simulink subsystem "rss_StrtUpElecAgCalcNeed"  (R2023a)
settings: Solver=VariableStepAuto  StartTime=0.0  StopTime=10.0  RelTol=1e-3
undefined symbols (not defined in the file): Cdbl_nElecAgSpdMaxVal, Cdbl_nElecAgSpdPeakVal, Cdbl_tiMedTaskSmpTi, ENM_MOTO_STATUS
libraries: lib_conversion x2, simulink x1, lib_discrete_time_integrator x1
settings Model: Creator=xiaoqiang.yuan  LastModifiedBy=xiaoqiang.yuan

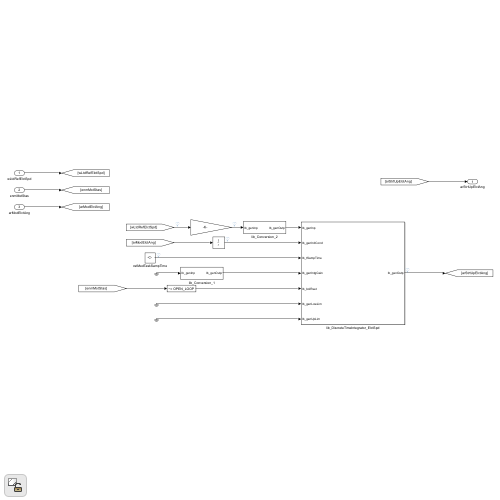
[thumbnail: Simulink's stored preview of the top-level diagram]
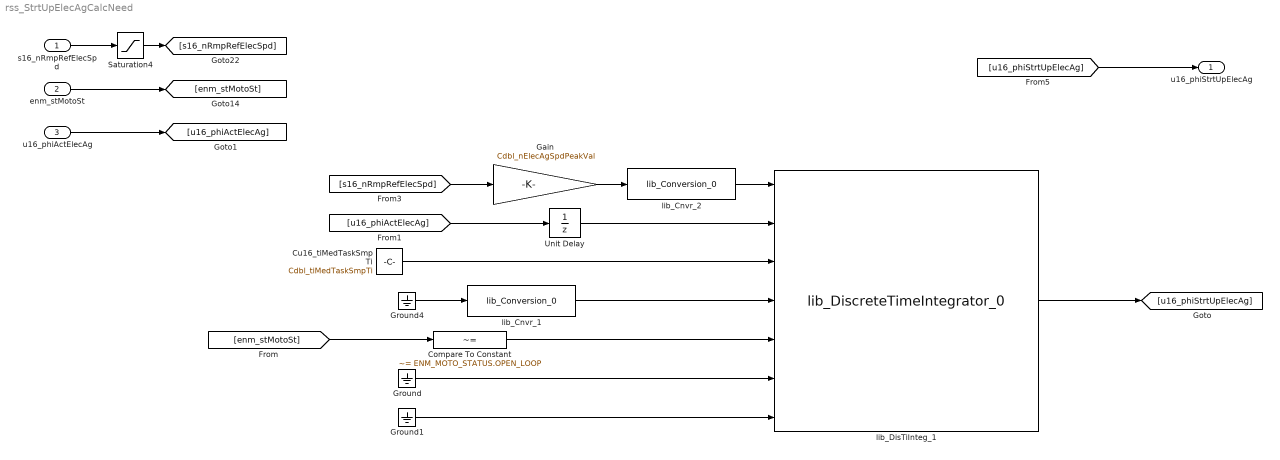
== system rss_StrtUpElecAgCalcNeed ==
  s16_nRmpRefElecSpd : Inport  OutDataTypeStr=dt_Standardize_s16p15b0
  enm_stMotoSt : Inport  Port=2  OutDataTypeStr=Enum: ENM_MOTO_STATUS  PortDimensions=1
  u16_phiActElecAg : Inport  Port=3  OutDataTypeStr=dt_RadAng_u16r15b0  PortDimensions=1
  Compare To Constant : simulink/Logic and Bit Operations/Compare To Constant  relop=~=  const=ENM_MOTO_STATUS.OPEN_LOOP  OutDataTypeStr=boolean
  Cu16_tiMedTaskSmpTi : Constant  Value=Cdbl_tiMedTaskSmpTi
  Gain : Gain  Gain=Cdbl_nElecAgSpdPeakVal  OutDataTypeStr=Inherit: Inherit via back propagation
  Ground : Ground
  Ground1 : Ground
  Ground4 : Ground
  Saturation4 : Saturate  UpperLimit=Cdbl_nElecAgSpdMaxVal  LowerLimit=-Cdbl_nElecAgSpdMaxVal
  Unit Delay : UnitDelay  SampleTime=-1  HasFrameUpgradeWarning=on
  lib_Cnvr_1 : lib_conversion/lib_Conversion_0  lb_parDataType=uint8  lb_parOutpMaxVal=[]  lb_parOutpMinVal=[]  lb_parSatFlag=off
  lib_Cnvr_2 : lib_conversion/lib_Conversion_0  lb_parDataType=fixdt(1,16)  lb_parOutpMaxVal=Cdbl_nElecAgSpdPeakVal  lb_parOutpMinVal=[]  RndMeth=Simplest  lb_parSatFlag=off
  lib_DisTiInteg_1 : lib_discrete_time_integrator/lib_DiscreteTimeIntegrator_0  lb_parMaxInpVal=Cdbl_nElecAgSpdMaxVal*Cdbl_nElecAgSpdPeakVal  lb_parMinInpVal=-Cdbl_nElecAgSpdMaxVal*Cdbl_nElecAgSpdPeakVal  lb_parMaxSampTime=double(Cdbl_tiMedTaskSmpTi)  lb_parMaxIntgGain=0  lb_parAccmDataTypeMode=Same of output  lb_parOutpDataType=dt_RadAng_u16r15b0  lb_parIntgScopMode=Angular signal  lb_parSatFlag=off
  u16_phiStrtUpElecAg : Outport  OutDataTypeStr=dt_RadAng_u16r15b0
  wires:
  [u16_phiStrtUpElecAg] -> u16_phiStrtUpElecAg/1
  Cu16_tiMedTaskSmpTi/1 -> lib_DisTiInteg_1/3
  lib_DisTiInteg_1/1 -> [u16_phiStrtUpElecAg]
  Ground4/1 -> lib_Cnvr_1/1
  enm_stMotoSt/1 -> [enm_stMotoSt]
  Ground/1 -> lib_DisTiInteg_1/6
  Compare To Constant/1 -> lib_DisTiInteg_1/5
  s16_nRmpRefElecSpd/1 -> Saturation4/1
  Ground1/1 -> lib_DisTiInteg_1/7
  lib_Cnvr_1/1 -> lib_DisTiInteg_1/4
  [enm_stMotoSt] -> Compare To Constant/1
  u16_phiActElecAg/1 -> [u16_phiActElecAg]
  Unit Delay/1 -> lib_DisTiInteg_1/2
  [u16_phiActElecAg] -> Unit Delay/1
  Gain/1 -> lib_Cnvr_2/1
  lib_Cnvr_2/1 -> lib_DisTiInteg_1/1
  [s16_nRmpRefElecSpd] -> Gain/1
  Saturation4/1 -> [s16_nRmpRefElecSpd]
